simulink model "discrete_bdot"  (R2024a)
settings: Solver=FixedStepAuto  StartTime=0.0  StopTime=17000  RelTol=1e-3
values from neighbouring files (symbols this model uses):
  Ib = [Ixx Ixy Izx ... (first row only)    [SatelliteMissionAnalysis2.m]    (also in dynamics_setup.m)
  Ibinv = Ib^-1    [dynamics_setup.m]
  K = 10^5    (= 100000)    [dynamics_setup.m]
  kick = [1; 2; 2]    [dynamics_setup.m]
  q0 = q0/norm(q0)    [dynamics_setup.m]
  Ts = 1    [dynamics_setup.m]
libraries: matrix_library x2, simulink x1
settings Model: Creator=Zargai  LastModifiedBy=Zargai
settings RTWCC: GenCodeOnly=on

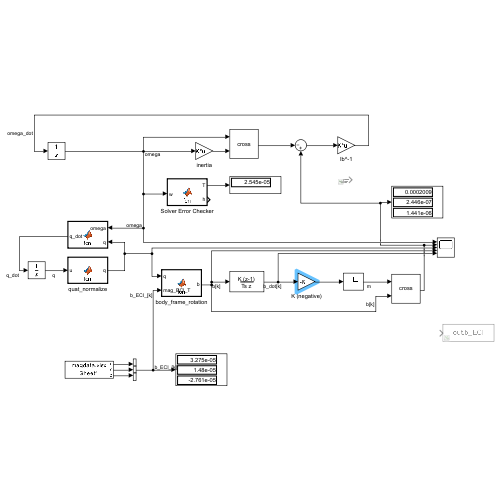
[thumbnail: Simulink's stored preview of the top-level diagram]
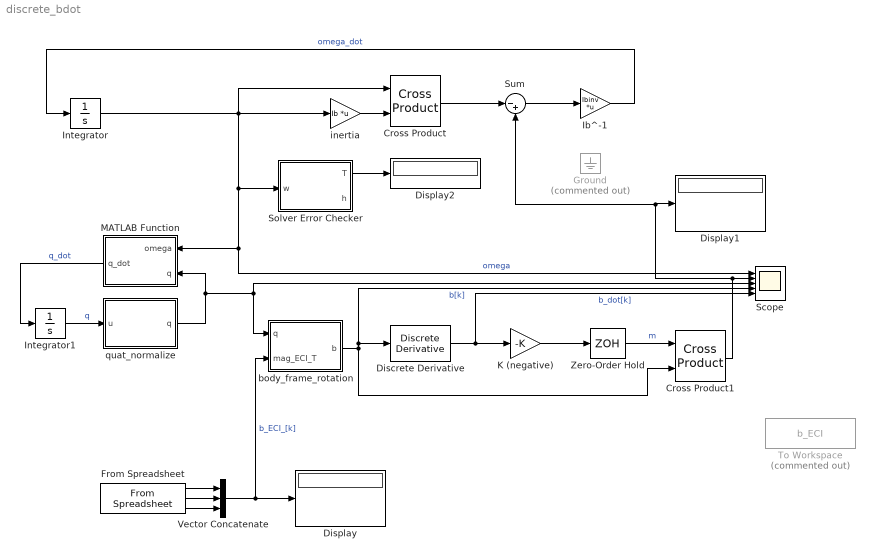
== system discrete_bdot ==
  Cross Product : matrix_library/Cross Product
  Cross Product1 : matrix_library/Cross Product
  Discrete Derivative : simulink/Discrete/Discrete Derivative  gainval=1.0  ICPrevScaledInput=0.0  OutMin=[]  OutMax=[]  OutDataType=fixdt(1, 16)  OutScaling=2^-10  DoSatur=off
  Display : Display
  Display1 : Display
  Display2 : Display
  From Spreadsheet : FromSpreadsheet  FileName=magdata.xlsx  SampleTime=Ts  ExtrapolationBeforeFirstDataPoint=Hold first value  InterpolationWithinTimeRange=Zero order hold  ExtrapolationAfterLastDataPoint=Hold last value
  Ground : Ground  Commented=on
  Ib^-1 : Gain  Gain=Ibinv  Multiplication=Matrix(K*u)
  Integrator : Integrator  InitialCondition=kick
  Integrator1 : Integrator  InitialCondition=q0
  K (negative) : Gain  Gain=-K
  MATLAB Function : MATLAB Function  TreatAsAtomicUnit=on
  Scope : Scope  NumInputPorts=5
  Solver Error Checker : MATLAB Function  TreatAsAtomicUnit=on
  Sum : Sum  Inputs=|-+
  To Workspace : ToWorkspace  Commented=on  VariableName=b_ECI  SaveFormat=Timeseries  SampleTime=-1
  Vector Concatenate : Concatenate  NumInputs=3
  Zero-Order Hold : ZeroOrderHold  SampleTime=Ts
  body_frame_rotation : MATLAB Function  TreatAsAtomicUnit=on
  inertia : Gain  Gain=Ib  Multiplication=Matrix(K*u)
  quat_normalize : MATLAB Function  TreatAsAtomicUnit=on
  wires:
  Integrator/1 -> inertia/1, Solver Error Checker/1(w), Scope/1, MATLAB Function/1(omega), Cross Product/1  "omega"
  MATLAB Function/1(q_dot) -> Integrator1/1  "q_dot"
  Integrator1/1 -> quat_normalize/1(u)  "q"
  Ib^-1/1 -> Integrator/1  "omega_dot"
  inertia/1 -> Cross Product/2
  Cross Product/1 -> Sum/1
  Sum/1 -> Ib^-1/1
  From Spreadsheet/1 -> Vector Concatenate/1
  From Spreadsheet/3 -> Vector Concatenate/3
  From Spreadsheet/2 -> Vector Concatenate/2
  quat_normalize/1(q) -> MATLAB Function/2(q), Scope/3, body_frame_rotation/1(q)
  Solver Error Checker/1(T) -> Display2/1
  Vector Concatenate/1 -> body_frame_rotation/2(mag_ECI_T), Display/1  "b_ECI_[k]"
  Discrete Derivative/1 -> K (negative)/1, Scope/5  "b_dot[k]"
  K (negative)/1 -> Zero-Order Hold/1
  body_frame_rotation/1(b) -> Scope/4, Discrete Derivative/1, Cross Product1/2  "b[k]"
  Zero-Order Hold/1 -> Cross Product1/1  "m"
  Cross Product1/1 -> Sum/2, Display1/1, Scope/2

== matlab function discrete_bdot/MATLAB Function ==
  data: omega input; q input; q_dot output
function q_dot = fcn(omega, q)

% Reference Crassidis Ch. 7.1

% skew = [0 -omega(3) omega(2);
%     omega(3) 0 -omega(1);
%     -omega(2) omega(1) 0];

% q_dot = .5* [-skew omega;
%     -omega' 0]* q;

q_dot = .5 * quat_cross_mult([omega; 0], q);

== matlab function discrete_bdot/quat_normalize ==
  data: u input; q output
function q = fcn(u)

q = u/norm(u);

== matlab function discrete_bdot/Solver Error Checker ==
  data: w input; T output; h output
function [T, h] = fcn(w)

Ixx = .03293;
Iyy = .13199;
Izz = .13943;
Ixy = .00005;
Iyz = -.00016;
Izx = -.00014;

Ib = [Ixx Ixy Izx;
    Ixy Iyy Iyz;
    Izx Iyz Izz];

T = w'*Ib*w;
h = norm(Ib*w);

== matlab function discrete_bdot/body_frame_rotation ==
  data: q input; b output; mag_ECI_T input
function b = fcn(q, mag_ECI_T)

bq = quat_cross_mult(q, quat_cross_mult( [mag_ECI_T; 0] , quat_inv(q))); % Embed mag_ECI into quat and Transform from ECI to Body frame
b = bq(1:3);
